simulink model "BG"  (R2014a)
settings: Solver=ode3  StartTime=0.0  StopTime=1  FixedStep=dt  MaxStep=dt  RelTol=1e-3
values from neighbouring files (symbols this model uses):
  a1 = .4    (= 0.4)    [parameters.m]
  a2 = .35    (= 0.35)    [parameters.m]
  a3 = .25    (= 0.25)    [parameters.m]
  aTc = 0.05    [parameters.m]
  dt = 1e-3    (= 0.001)    [parameters.m]
  g = 1    [parameters.m]
  K = 1    [parameters.m]
  mTc = 0.01    [parameters.m]
  OP1_0 = [ax1_0 ay1_0 0]    [parameters.m]
  OP2_0 = OP1_0 + P1P2_0    [parameters.m]
  OP3_0 = OP2_0 + P2P3_0    [parameters.m]
  OT = [xf yf 0]    [animation.m]    (also in parameters.m = [0.5 0.5 0])
  OT_cercle = [0.6 0.55 0]    [parameters.m]
  p1 = w2 + w3    (= 3)    [parameters.m]
  P1P2_0 = [ax2_0 ay2_0 0]    [parameters.m]
  p2 = w1 + w3    (= 4)    [parameters.m]
  P2P3_0 = [ax3_0 ay3_0 0]    [parameters.m]
  p3 = w2 + w1    (= 5)    [parameters.m]
  tau = 0.001    [parameters.m]
  theta1_0 = zero_vector    [parameters.m]
  theta2_0 = zero_vector    [parameters.m]
  theta3_0 = zero_vector    [parameters.m]
  Vmax = 30    [parameters.m]
  w1 = 3    [parameters.m]
  w2 = 2    [parameters.m]
  w3 = 1    [parameters.m]
  zero_vector = [0 0 0]    [parameters.m]
libraries: vrlib x9, simulink x1
(part 2 of 4)

== system BG/CNS/ Striosom//SNc2/Optimiseur1 ==
  v : Inport
  a1 : Inport  Port=2
  a2 : Inport  Port=3
  a3 : Inport  Port=4
  "                                                                                                    " : Sum  Inputs=+--
  B1 : Subsystem
  B2 : Subsystem
  Gain : Gain  Gain=w1
  Gain1 : Gain  Gain=w2
  Gamma1 : Subsystem
  Gamma2 : Subsystem
  lambda : Subsystem
  matrix_vector_multiplication : Subsystem
  matrix_vector_multiplication1 : Subsystem
  x : Scope
  v1 : Outport
  v2 : Outport  Port=2
  v3 : Outport  Port=3
  wires:
  v/1 -> "                                                                                                    "/1, matrix_vector_multiplication1/1(v1), matrix_vector_multiplication/1(v1), B2/1(v), B1/1(v), lambda/1(v)
  a1/1 -> B1/4(a1), lambda/2(a1)
  a2/1 -> B2/4(a2), lambda/3(a2)
  a3/1 -> B2/5(a3), B1/5(a3), lambda/4(a3)
  lambda/1(lambda1) -> B1/2(lambda1)
  lambda/3(lambda3) -> B1/3(lambda3), B2/3(lambda3)
  lambda/2(lamda2) -> B2/2(lambda2)
  B1/1(b11) -> Gamma2/5(b11_2), Gamma1/1(b11_1)
  B1/2(b12) -> Gamma2/6(b12_2), Gamma1/2(b12_1)
  B1/3(b21) -> Gamma2/7(b21_2), Gamma1/3(b21_1)
  B1/4(b22) -> Gamma2/8(b22_2), Gamma1/4(b22_1)
  B2/1(b11) -> Gamma1/5(b11_2), Gamma2/1(b11_1)
  B2/2(b12) -> Gamma1/6(b12_2), Gamma2/2(b12_1)
  B2/3(b21) -> Gamma1/7(b21_2), Gamma2/3(b21_1)
  B2/4(b22) -> Gamma2/4(b22_1), Gamma1/8(b22_2)
  Gamma1/1(gamma11) -> matrix_vector_multiplication/2(a11)
  Gamma1/2(gamma12) -> matrix_vector_multiplication/3(a12)
  Gamma1/3(gamma21) -> matrix_vector_multiplication/4(a21)
  Gamma1/4(gamma22) -> matrix_vector_multiplication/5(a22)
  Gamma2/1(gamma11) -> matrix_vector_multiplication1/2(a11)
  Gamma2/2(gamma12) -> matrix_vector_multiplication1/3(a12)
  Gamma2/3(gamma21) -> matrix_vector_multiplication1/4(a21)
  Gamma2/4(gamma22) -> matrix_vector_multiplication1/5(a22)
  matrix_vector_multiplication/1(vec_out) -> Gain/1
  matrix_vector_multiplication1/1(vec_out) -> Gain1/1
  "                                                                                                    "/1 -> v3/1
  Gain/1 -> x/1, "                                                                                                    "/2, v1/1
  Gain1/1 -> "                                                                                                    "/3, v2/1

== system BG/CNS/ Striosom//SNc2/derivative ==
  x : Inport
  Add : Sum  Inputs=+-
  Delay : Delay  DelayLength=1  InitialCondition=zero_vector
  Gain : Gain  Gain=1/dt
  z : Outport
  wires:
  Add/1 -> Gain/1
  x/1 -> Delay/1, Add/1
  Delay/1 -> Add/2
  Gain/1 -> z/1

== system BG/CNS/ Striosom//SNc2/derivative1 ==
  x : Inport
  Add : Sum  Inputs=+-
  Delay : Delay  DelayLength=1  InitialCondition=zero_vector
  Gain : Gain  Gain=1/dt
  z : Outport
  wires:
  Add/1 -> Gain/1
  x/1 -> Delay/1, Add/1
  Delay/1 -> Add/2
  Gain/1 -> z/1

== system BG/CNS/ Striosom//SNc2/derivative2 ==
  x : Inport
  Add : Sum  Inputs=+-
  Delay : Delay  DelayLength=1  InitialCondition=zero_vector
  Gain : Gain  Gain=1/dt
  z : Outport
  wires:
  Add/1 -> Gain/1
  x/1 -> Delay/1, Add/1
  Delay/1 -> Add/2
  Gain/1 -> z/1

== system BG/CNS/ Striosom//SNc2/vector_scope1 ==
  In_vec : Inport
  Demux : Demux  Outputs=3
  x : Scope
  y : Scope
      settings: SaveName=ScopeData2
  z : Scope
      settings: SaveName=ScopeData3
  wires:
  In_vec/1 -> Demux/1
  Demux/1 -> x/1
  Demux/2 -> y/1
  Demux/3 -> z/1

== system BG/CNS/ Striosom//SNc2/vector_scope2 ==
  In_vec : Inport
  Demux : Demux  Outputs=3
  x : Scope
  y : Scope
      settings: SaveName=ScopeData2
  z : Scope
      settings: SaveName=ScopeData3
  wires:
  In_vec/1 -> Demux/1
  Demux/1 -> x/1
  Demux/2 -> y/1
  Demux/3 -> z/1

== system BG/CNS/ Striosom//SNc2/vector_scope3 ==
  In_vec : Inport
  Demux : Demux  Outputs=3
  x : Scope
  y : Scope
      settings: SaveName=ScopeData2
  z : Scope
      settings: SaveName=ScopeData3
  wires:
  In_vec/1 -> Demux/1
  Demux/1 -> x/1
  Demux/2 -> y/1
  Demux/3 -> z/1

== system BG/CNS/Circular movement/1//(T*s+1) ==
  x : Inport
  Add : Sum  Inputs=+-
  Add1 : Sum
  Delay : Delay  DelayLength=1  InitialCondition=OP3_0
  Gain : Gain  Gain=dt
  Gain2 : Gain  Gain=1/0.01
  z : Outport
  wires:
  Add/1 -> Gain/1
  Delay/1 -> Add1/2, Add/2
  Gain/1 -> Gain2/1
  x/1 -> Add/1
  Add1/1 -> z/1, Delay/1
  Gain2/1 -> Add1/1

== system BG/CNS/Circular movement/1//(T*s+1)1 ==
  x : Inport
  Add : Sum  Inputs=+-
  Add1 : Sum
  Delay : Delay  DelayLength=1  InitialCondition=OP3_0
  Gain : Gain  Gain=dt
  Gain2 : Gain  Gain=1/0.001
  z : Outport
  wires:
  Add/1 -> Gain/1
  Delay/1 -> Add1/2, Add/2
  Gain/1 -> Gain2/1
  x/1 -> Add/1
  Add1/1 -> z/1, Delay/1
  Gain2/1 -> Add1/1

== system BG/CNS/Circular movement/1//(T*s+1)2 ==
  x : Inport
  Add : Sum  Inputs=+-
  Add1 : Sum
  Delay : Delay  DelayLength=1  InitialCondition=OP3_0
  Gain : Gain  Gain=dt
  Gain2 : Gain  Gain=1/0.002
  z : Outport
  wires:
  Add/1 -> Gain/1
  Delay/1 -> Add1/2, Add/2
  Gain/1 -> Gain2/1
  x/1 -> Add/1
  Add1/1 -> z/1, Delay/1
  Gain2/1 -> Add1/1

== system BG/CNS/Circular movement/Theta_point1 ==
  In_vec : Inport
  Demux : Demux  Outputs=3
  x : Scope
      settings: YMin=0.74125  YMax=0.745
  y : Scope
      settings: YMin=0.59325  YMax=0.5965  SaveName=ScopeData2
  z : Scope
      settings: SaveName=ScopeData3
  wires:
  In_vec/1 -> Demux/1
  Demux/2 -> y/1
  Demux/3 -> z/1
  Demux/1 -> x/1

== system BG/CNS/Circular movement/Theta_point2 ==
  In_vec : Inport
  Demux : Demux  Outputs=3
  x : Scope
      settings: YMin=0.74125  YMax=0.745
  y : Scope
      settings: YMin=0.45  YMax=0.75  SaveName=ScopeData2
  z : Scope
      settings: SaveName=ScopeData3
  wires:
  In_vec/1 -> Demux/1
  Demux/2 -> y/1
  Demux/3 -> z/1
  Demux/1 -> x/1

== system BG/CNS/Circular movement/Theta_point3 ==
  In_vec : Inport
  Demux : Demux  Outputs=3
  x : Scope
      settings: YMin=0.74125  YMax=0.745
  y : Scope
      settings: YMin=0.59325  YMax=0.5965  SaveName=ScopeData2
  z : Scope
      settings: SaveName=ScopeData3
  wires:
  In_vec/1 -> Demux/1
  Demux/2 -> y/1
  Demux/3 -> z/1
  Demux/1 -> x/1

== system BG/CNS/Cortex M1/derivative ==
  x : Inport
  Add : Sum  Inputs=+-
  Delay : Delay  DelayLength=1  InitialCondition=zero_vector
  Gain : Gain  Gain=1/dt
  z : Outport
  wires:
  Add/1 -> Gain/1
  x/1 -> Delay/1, Add/1
  Delay/1 -> Add/2
  Gain/1 -> z/1

== system BG/CNS/Cortex M1/derivative1 ==
  x : Inport
  Add : Sum  Inputs=+-
  Delay : Delay  DelayLength=1  InitialCondition=zero_vector
  Gain : Gain  Gain=1/dt
  z : Outport
  wires:
  Add/1 -> Gain/1
  x/1 -> Delay/1, Add/1
  Delay/1 -> Add/2
  Gain/1 -> z/1

== system BG/CNS/Cortex M1/derivative2 ==
  x : Inport
  Add : Sum  Inputs=+-
  Delay : Delay  DelayLength=1  InitialCondition=zero_vector
  Gain : Gain  Gain=1/dt
  z : Outport
  wires:
  Add/1 -> Gain/1
  x/1 -> Delay/1, Add/1
  Delay/1 -> Add/2
  Gain/1 -> z/1

== system BG/CNS/GPe/1//(sigma*s+1) ==
  x : Inport
  Add : Sum  Inputs=+-
  Add1 : Sum
  Delay : Delay  DelayLength=1  InitialCondition=zero_vector
  Gain : Gain  Gain=dt
  Gain1 : Gain  Gain=0.9999999
  Gain2 : Gain  Gain=1/tau
  z : Outport
  wires:
  Add/1 -> Gain/1
  Gain1/1 -> Add1/2, Add/2
  Delay/1 -> Gain1/1
  Gain/1 -> Gain2/1
  x/1 -> Add/1
  Add1/1 -> z/1, Delay/1
  Gain2/1 -> Add1/1

== system BG/CNS/GPe/1//(sigma*s+1)1 ==
  x : Inport
  Add : Sum  Inputs=+-
  Add1 : Sum
  Delay : Delay  DelayLength=1  InitialCondition=zero_vector
  Gain : Gain  Gain=dt
  Gain1 : Gain  Gain=0.9999999
  Gain2 : Gain  Gain=1/tau
  z : Outport
  wires:
  Add/1 -> Gain/1
  Gain1/1 -> Add1/2, Add/2
  Delay/1 -> Gain1/1
  Gain/1 -> Gain2/1
  x/1 -> Add/1
  Add1/1 -> z/1, Delay/1
  Gain2/1 -> Add1/1

== system BG/CNS/GPe/1//(sigma*s+1)2 ==
  x : Inport
  Add : Sum  Inputs=+-
  Add1 : Sum
  Delay : Delay  DelayLength=1  InitialCondition=zero_vector
  Gain : Gain  Gain=dt
  Gain1 : Gain  Gain=0.9999999
  Gain2 : Gain  Gain=1/tau
  z : Outport
  wires:
  Add/1 -> Gain/1
  Gain1/1 -> Add1/2, Add/2
  Delay/1 -> Gain1/1
  Gain/1 -> Gain2/1
  x/1 -> Add/1
  Add1/1 -> z/1, Delay/1
  Gain2/1 -> Add1/1

== system BG/CNS/GPe/Theta_point4 ==
  In_vec : Inport
  Demux : Demux  Outputs=3
  x : Scope
  y : Scope
      settings: SaveName=ScopeData2
  z : Scope
      settings: TimeRange=2  SaveName=ScopeData3
  wires:
  In_vec/1 -> Demux/1
  Demux/1 -> x/1
  Demux/2 -> y/1
  Demux/3 -> z/1

== system BG/CNS/Gains  (STR1)/Normaliser ==
  PS1 : Inport
  PS2 : Inport  Port=2
  PS3 : Inport  Port=3
  PV1 : Inport  Port=4
  PV2 : Inport  Port=5
  PV 3 : Inport  Port=6
  "                  " : Sum
  "                                  " : Gain  Gain=1/(a1^2)
  "                                       " : Sum
  "                                                                    " : Gain  Gain=1/(a2^2)
  "                                                                                     " : Sum
  "                                                                                                               " : Gain  Gain=1/(a3^2)
  PS1+PV1 : Outport
  PS2+PV2 : Outport  Port=2
  PS3+PV3 : Outport  Port=3
  wires:
  "                  "/1 -> "                                                                    "/1
  PV2/1 -> "                  "/2
  PS2/1 -> "                  "/1
  "                                                                    "/1 -> PS2+PV2/1
  "                                  "/1 -> PS1+PV1/1
  "                                                                                     "/1 -> "                                  "/1
  PV1/1 -> "                                                                                     "/2
  PS1/1 -> "                                                                                     "/1
  "                                       "/1 -> "                                                                                                               "/1
  "                                                                                                               "/1 -> PS3+PV3/1
  PV 3/1 -> "                                       "/2
  PS3/1 -> "                                       "/1

== system BG/CNS/Positionof segments Forward Kinematics/unit_vec ==
  vec1 : Inport
  Divide : Product  Inputs=*/
  Dot Product3 : DotProduct  InputSameDT=on  OutDataTypeStr=Inherit: Inherit via internal rule
  Sqrt : Sqrt  SaturateOnIntegerOverflow=on
  vec2 : Outport
  wires:
  vec1/1 -> Divide/1, Dot Product3/2, Dot Product3/1
  Dot Product3/1 -> Sqrt/1
  Sqrt/1 -> Divide/2
  Divide/1 -> vec2/1

== system BG/CNS/Positionof segments Forward Kinematics/unit_vec1 ==
  vec1 : Inport
  Divide : Product  Inputs=*/
  Dot Product3 : DotProduct  InputSameDT=on  OutDataTypeStr=Inherit: Inherit via internal rule
  Sqrt : Sqrt  SaturateOnIntegerOverflow=on
  vec2 : Outport
  wires:
  vec1/1 -> Divide/1, Dot Product3/2, Dot Product3/1
  Dot Product3/1 -> Sqrt/1
  Sqrt/1 -> Divide/2
  Divide/1 -> vec2/1

== system BG/CNS/Positionof segments Forward Kinematics/unit_vec2 ==
  vec1 : Inport
  Divide : Product  Inputs=*/
  Dot Product3 : DotProduct  InputSameDT=on  OutDataTypeStr=Inherit: Inherit via internal rule
  Sqrt : Sqrt  SaturateOnIntegerOverflow=on
  vec2 : Outport
  wires:
  vec1/1 -> Divide/1, Dot Product3/2, Dot Product3/1
  Dot Product3/1 -> Sqrt/1
  Sqrt/1 -> Divide/2
  Divide/1 -> vec2/1

== system BG/CNS/Reaching/1//(T*s+1) ==
  x : Inport
  Add : Sum  Inputs=+-
  Add1 : Sum
  Delay : Delay  DelayLength=1  InitialCondition=OP3_0
  Gain : Gain  Gain=dt
  Gain2 : Gain  Gain=1/0.01
  z : Outport
  wires:
  Add/1 -> Gain/1
  Delay/1 -> Add1/2, Add/2
  Gain/1 -> Gain2/1
  x/1 -> Add/1
  Add1/1 -> z/1, Delay/1
  Gain2/1 -> Add1/1

== system BG/CNS/Reaching/Theta_point1 ==
  In_vec : Inport
  Demux : Demux  Outputs=3
  x : Scope
  y : Scope
      settings: SaveName=ScopeData2
  z : Scope
      settings: SaveName=ScopeData3
  wires:
  In_vec/1 -> Demux/1
  Demux/1 -> x/1
  Demux/2 -> y/1
  Demux/3 -> z/1

== system BG/CNS/Reaching/derivative ==
  x : Inport
  Add : Sum  Inputs=+-
  Delay : Delay  DelayLength=1  InitialCondition=OP3_0
  Gain : Gain  Gain=1/dt
  z : Outport
  wires:
  Add/1 -> Gain/1
  x/1 -> Delay/1, Add/1
  Delay/1 -> Add/2
  Gain/1 -> z/1

== system BG/CNS/Reaching/vitesse ==
  In_vec : Inport
  Demux : Demux  Outputs=3
  x : Scope
      settings: TimeRange=1.4  YMin=-90  YMax=0
  y : Scope
      settings: SaveName=ScopeData2
  z : Scope
      settings: SaveName=ScopeData3
  wires:
  In_vec/1 -> Demux/1
  Demux/1 -> x/1
  Demux/2 -> y/1
  Demux/3 -> z/1

== system BG/CNS/STN/1//(sigma*s+1) ==
  x : Inport
  Add : Sum  Inputs=+-
  Add1 : Sum
  Delay : Delay  DelayLength=1  InitialCondition=0
  Gain : Gain  Gain=dt
  Gain1 : Gain  Gain=0.9999999
  Gain2 : Gain  Gain=1/mTc
  z : Outport
  wires:
  Add/1 -> Gain/1
  Gain1/1 -> Add1/2, Add/2
  Delay/1 -> Gain1/1
  Gain/1 -> Gain2/1
  x/1 -> Add/1
  Gain2/1 -> Add1/1
  Add1/1 -> z/1, Delay/1

== system BG/CNS/STN/1//(sigma*s+1)1 ==
  x : Inport
  Add : Sum  Inputs=+-
  Add1 : Sum
  Delay : Delay  DelayLength=1  InitialCondition=0
  Gain : Gain  Gain=dt
  Gain1 : Gain  Gain=0.9999999
  Gain2 : Gain  Gain=1/mTc
  z : Outport
  wires:
  Add/1 -> Gain/1
  Gain1/1 -> Add1/2, Add/2
  Delay/1 -> Gain1/1
  Gain/1 -> Gain2/1
  x/1 -> Add/1
  Gain2/1 -> Add1/1
  Add1/1 -> z/1, Delay/1

== system BG/CNS/STN/1//(sigma*s+1)2 ==
  x : Inport
  Add : Sum  Inputs=+-
  Add1 : Sum
  Delay : Delay  DelayLength=1  InitialCondition=0
  Gain : Gain  Gain=dt
  Gain1 : Gain  Gain=0.9999999
  Gain2 : Gain  Gain=1/mTc
  z : Outport
  wires:
  Add/1 -> Gain/1
  Gain1/1 -> Add1/2, Add/2
  Delay/1 -> Gain1/1
  Gain/1 -> Gain2/1
  x/1 -> Add/1
  Gain2/1 -> Add1/1
  Add1/1 -> z/1, Delay/1

== system BG/CNS/STN/s//(Ts+1) ==
  In1 : Inport
  1/(sigma*s+1) : Subsystem  TreatAsAtomicUnit=on
  derivative : Subsystem  TreatAsAtomicUnit=on
  Out1 : Outport
  wires:
  In1/1 -> 1/(sigma*s+1)/1(x)
  1/(sigma*s+1)/1(z) -> derivative/1(x)
  derivative/1(z) -> Out1/1

== system BG/CNS/STN/s//(Ts+1)2 ==
  In1 : Inport
  1/(sigma*s+1) : Subsystem  TreatAsAtomicUnit=on
  derivative : Subsystem  TreatAsAtomicUnit=on
  Out1 : Outport
  wires:
  In1/1 -> 1/(sigma*s+1)/1(x)
  1/(sigma*s+1)/1(z) -> derivative/1(x)
  derivative/1(z) -> Out1/1

== system BG/CNS/STN/s//(Ts+1)3 ==
  In1 : Inport
  1/(sigma*s+1) : Subsystem  TreatAsAtomicUnit=on
  derivative : Subsystem  TreatAsAtomicUnit=on
  Out1 : Outport
  wires:
  In1/1 -> 1/(sigma*s+1)/1(x)
  1/(sigma*s+1)/1(z) -> derivative/1(x)
  derivative/1(z) -> Out1/1

== system BG/CNS/Thalamus/Theta_point1 ==
  In_vec : Inport
  Demux : Demux  Outputs=3
  x : Scope
  y : Scope
      settings: SaveName=ScopeData2
  z : Scope
      settings: SaveName=ScopeData3
  wires:
  In_vec/1 -> Demux/1
  Demux/1 -> x/1
  Demux/2 -> y/1
  Demux/3 -> z/1

== system BG/CNS/Vector Product  (STR1)/Integrateur ==
  In1 : Inport
  " " : Delay  DelayLength=1  InitialCondition=zero_vector
  "  " : Sum
  "        " : Gain  Gain=dt
  Out1 : Outport
  wires:
  "        "/1 -> "  "/1
  " "/1 -> "  "/2
  In1/1 -> "        "/1
  "  "/1 -> " "/1, Out1/1

== system BG/CNS/Vector Product  (STR1)/Integrateur1 ==
  In1 : Inport
  " " : Delay  DelayLength=1  InitialCondition=zero_vector
  "  " : Sum
  "        " : Gain  Gain=dt
  Out1 : Outport
  wires:
  "        "/1 -> "  "/1
  " "/1 -> "  "/2
  In1/1 -> "        "/1
  "  "/1 -> " "/1, Out1/1

== system BG/CNS/Vector Product  (STR1)/Integrateur2 ==
  In1 : Inport
  " " : Delay  DelayLength=1  InitialCondition=zero_vector
  "  " : Sum
  "        " : Gain  Gain=dt
  Out1 : Outport
  wires:
  "        "/1 -> "  "/1
  " "/1 -> "  "/2
  In1/1 -> "        "/1
  "  "/1 -> " "/1, Out1/1

== system BG/CNS/ Striosom//SNc2/Optimiseur/B1 ==
  v : Inport
  lambda1 : Inport  Port=2
  lambda3 : Inport  Port=3
  a1 : Inport  Port=4
  a3 : Inport  Port=5
  Subsystem : Subsystem
  inverse_matrix : Subsystem
  vector_in_matrix_out : Subsystem
  b11 : Outport
  b12 : Outport  Port=2
  b21 : Outport  Port=3
  b22 : Outport  Port=4
  wires:
  vector_in_matrix_out/3(a21_out) -> inverse_matrix/3(a21)
  vector_in_matrix_out/1(a11_out) -> inverse_matrix/1(a11)
  vector_in_matrix_out/4(a22_out) -> inverse_matrix/4(a22)
  vector_in_matrix_out/2(a12_out) -> inverse_matrix/2(a12)
  lambda3/1 -> Subsystem/3(lambda3)
  inverse_matrix/3(a21_out) -> Subsystem/7(In7)
  a1/1 -> Subsystem/2(a1)
  a3/1 -> Subsystem/4(a3)
  v/1 -> vector_in_matrix_out/1(v1), vector_in_matrix_out/2(v2), Subsystem/8(In8)
  Subsystem/4(b22) -> b22/1
  Subsystem/3(b21) -> b21/1
  inverse_matrix/2(a12_out) -> Subsystem/6(In6)
  inverse_matrix/4(a22_out) -> Subsystem/9(In9)
  inverse_matrix/1(a11_out) -> Subsystem/5(In5)
  lambda1/1 -> Subsystem/1(lambda1)
  Subsystem/2(b12) -> b12/1
  Subsystem/1(b11) -> b11/1

== system BG/CNS/ Striosom//SNc2/Optimiseur/B2 ==
  v : Inport
  lambda2 : Inport  Port=2
  lambda3 : Inport  Port=3
  a2 : Inport  Port=4
  a3 : Inport  Port=5
  Subsystem : Subsystem
  inverse_matrix : Subsystem
  vector_in_matrix_out : Subsystem
  b11 : Outport
  b12 : Outport  Port=2
  b21 : Outport  Port=3
  b22 : Outport  Port=4
  wires:
  vector_in_matrix_out/3(a21_out) -> inverse_matrix/3(a21)
  vector_in_matrix_out/1(a11_out) -> inverse_matrix/1(a11)
  vector_in_matrix_out/4(a22_out) -> inverse_matrix/4(a22)
  vector_in_matrix_out/2(a12_out) -> inverse_matrix/2(a12)
  lambda3/1 -> Subsystem/3(lambda3)
  inverse_matrix/3(a21_out) -> Subsystem/7(In7)
  a2/1 -> Subsystem/2(a1)
  a3/1 -> Subsystem/4(a3)
  v/1 -> vector_in_matrix_out/1(v1), vector_in_matrix_out/2(v2), Subsystem/8(In8)
  Subsystem/4(b22) -> b22/1
  Subsystem/3(b21) -> b21/1
  inverse_matrix/2(a12_out) -> Subsystem/6(In6)
  inverse_matrix/4(a22_out) -> Subsystem/9(In9)
  inverse_matrix/1(a11_out) -> Subsystem/5(In5)
  lambda2/1 -> Subsystem/1(lambda1)
  Subsystem/2(b12) -> b12/1
  Subsystem/1(b11) -> b11/1

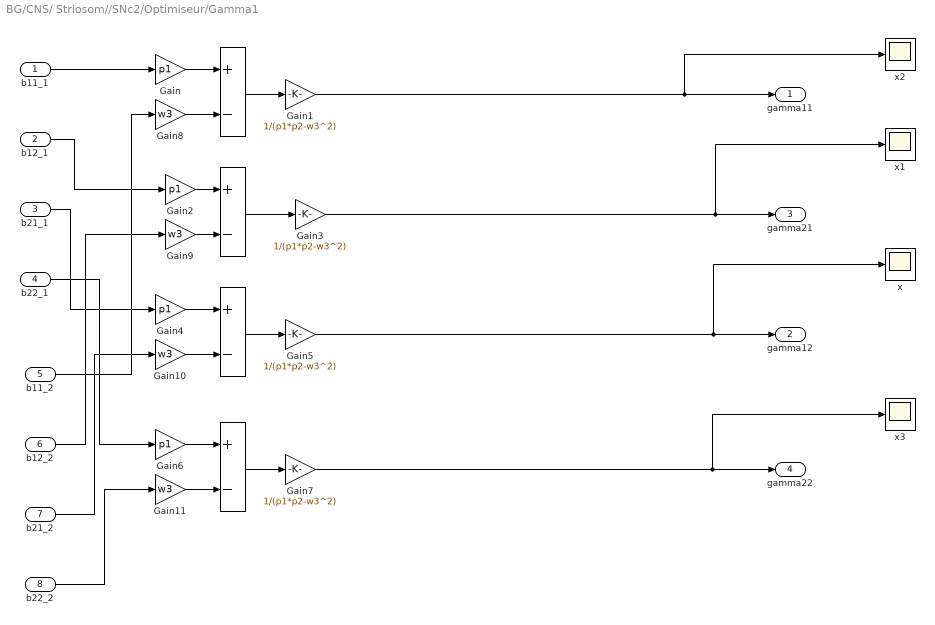
== system BG/CNS/ Striosom//SNc2/Optimiseur/Gamma1 ==
  b11_1 : Inport
  b12_1 : Inport  Port=2
  b21_1 : Inport  Port=3
  b22_1 : Inport  Port=4
  b11_2 : Inport  Port=5
  b12_2 : Inport  Port=6
  b21_2 : Inport  Port=7
  b22_2 : Inport  Port=8
  "                                                                                        " : Sum  Inputs=+-
  "                                                                                                " : Sum  Inputs=+-
  "                                                                                                  " : Sum  Inputs=+-
  "                                                                                                       " : Sum  Inputs=+-
  Gain{,2,4,6} (4 alike) : Gain  Gain=p1
  Gain{1,3,5,7} (4 alike) : Gain  Gain=1/(p1*p2-w3^2)
  Gain{8..11} (4 alike) : Gain  Gain=w3
  x{,1..3} (4 alike) : Scope
      x settings: YMin=-0.0001  YMax=0.0001  SaveName=ScopeData13
      x1 settings: YMin=-0.00045  YMax=0.0004  SaveName=ScopeData14
      x2 settings: YMin=-0.34905  YMax=-0.3486  SaveName=ScopeData15
      x3 settings: YMin=-0.348975  YMax=-0.348775  SaveName=ScopeData16
  gamma11 : Outport
  gamma12 : Outport  Port=2
  gamma21 : Outport  Port=3
  gamma22 : Outport  Port=4
  wires:
  b22_1/1 -> Gain6/1
  b21_1/1 -> Gain4/1
  b22_2/1 -> Gain11/1
  b11_1/1 -> Gain/1
  "                                                                                        "/1 -> Gain7/1
  "                                                                                                "/1 -> Gain5/1
  Gain6/1 -> "                                                                                        "/1
  Gain4/1 -> "                                                                                                "/1
  b21_2/1 -> Gain10/1
  b11_2/1 -> Gain8/1
  "                                                                                                       "/1 -> Gain1/1
  "                                                                                                  "/1 -> Gain3/1
  b12_2/1 -> Gain9/1
  Gain2/1 -> "                                                                                                  "/1
  b12_1/1 -> Gain2/1
  Gain/1 -> "                                                                                                       "/1
  Gain1/1 -> x2/1, gamma11/1
  Gain3/1 -> x1/1, gamma21/1
  Gain7/1 -> x3/1, gamma22/1
  Gain5/1 -> x/1, gamma12/1
  Gain8/1 -> "                                                                                                       "/2
  Gain9/1 -> "                                                                                                  "/2
  Gain10/1 -> "                                                                                                "/2
  Gain11/1 -> "                                                                                        "/2

== system BG/CNS/ Striosom//SNc2/Optimiseur/Gamma2 ==
  b11_1 : Inport
  b12_1 : Inport  Port=2
  b21_1 : Inport  Port=3
  b22_1 : Inport  Port=4
  b11_2 : Inport  Port=5
  b12_2 : Inport  Port=6
  b21_2 : Inport  Port=7
  b22_2 : Inport  Port=8
  "                                                                                        " : Sum
  "                                                                                                " : Sum
  "                                                                                                  " : Sum
  "                                                                                                       " : Sum
  Gain{1,3,5,8} (4 alike) : Gain  Gain=1/(w3*(p1*p2-w3^2))
  Gain{9..12} (4 alike) : Gain  Gain=w3*p2
  Gain{2,4,6..7} (4 alike) : Gain  Gain=(1-p1*p2)
  gamma11 : Outport
  gamma12 : Outport  Port=2
  gamma21 : Outport  Port=3
  gamma22 : Outport  Port=4
  wires:
  b22_1/1 -> Gain6/1
  b21_1/1 -> Gain4/1
  b22_2/1 -> Gain12/1
  b11_1/1 -> Gain7/1
  "                                                                                        "/1 -> Gain5/1
  "                                                                                                "/1 -> Gain8/1
  Gain6/1 -> "                                                                                        "/1
  Gain4/1 -> "                                                                                                "/1
  b21_2/1 -> Gain11/1
  b11_2/1 -> Gain9/1
  "                                                                                                       "/1 -> Gain1/1
  "                                                                                                  "/1 -> Gain3/1
  b12_2/1 -> Gain10/1
  Gain2/1 -> "                                                                                                  "/1
  b12_1/1 -> Gain2/1
  Gain7/1 -> "                                                                                                       "/1
  Gain1/1 -> gamma11/1
  Gain3/1 -> gamma21/1
  Gain5/1 -> gamma22/1
  Gain8/1 -> gamma12/1
  Gain9/1 -> "                                                                                                       "/2
  Gain10/1 -> "                                                                                                  "/2
  Gain11/1 -> "                                                                                                "/2
  Gain12/1 -> "                                                                                        "/2

== system BG/CNS/ Striosom//SNc2/Optimiseur/lambda ==
  v : Inport
  a1 : Inport  Port=2
  a2 : Inport  Port=3
  a3 : Inport  Port=4
  alpha : Subsystem
  d=V^T(VV^T)^-1V : Subsystem
  lambda : Subsystem
  other_aux_variables : Subsystem
  producing_dot_productions : Subsystem
  x : Scope
      settings: YMin=-0.7  YMax=1  SaveName=ScopeData12
  lambda1 : Outport
  lamda2 : Outport  Port=2
  lambda3 : Outport  Port=3
  wires:
  other_aux_variables/1(beta) -> lambda/1(beta)
  other_aux_variables/2(delta1) -> lambda/2(delta1)
  other_aux_variables/3(delta2) -> lambda/3(delta2)
  a2/1 -> producing_dot_productions/3(a2)
  producing_dot_productions/8(b23) -> lambda/8(b23), other_aux_variables/5(b23)
  a3/1 -> producing_dot_productions/4(a3)
  producing_dot_productions/9(b33) -> lambda/9(b33), other_aux_variables/6(b33)
  producing_dot_productions/6(b13) -> other_aux_variables/3(b13), lambda/7(b13)
  alpha/3(alpha3) -> lambda/6(alpha3), other_aux_variables/9(alpha3)
  producing_dot_productions/1(c1) -> alpha/2(c1)
  producing_dot_productions/5(b12) -> other_aux_variables/2(b12)
  v/1 -> producing_dot_productions/1(v), d=V^T(VV^T)^-1V/1(In1)
  other_aux_variables/5(gessi2) -> lambda/5(gessi2)
  producing_dot_productions/7(b22) -> other_aux_variables/4(b22)
  producing_dot_productions/4(b11) -> other_aux_variables/1(b11)
  alpha/2(alpha2) -> other_aux_variables/8(alpha2)
  alpha/1(alpha1) -> other_aux_variables/7(alpha1)
  other_aux_variables/4(gessi1) -> lambda/4(gessi1)
  producing_dot_productions/3(c3) -> alpha/4(c3)
  a1/1 -> producing_dot_productions/2(a1)
  d=V^T(VV^T)^-1V/1(d) -> alpha/1(d)
  producing_dot_productions/2(c2) -> alpha/3(c2)
  lambda/1(lambda1) -> lambda1/1
  lambda/3(lambda3) -> lambda3/1
  lambda/2(lambda2) -> lamda2/1

== system BG/CNS/ Striosom//SNc2/Optimiseur/matrix_vector_multiplication ==
  v1 : Inport
  a11 : Inport  Port=2
  a12 : Inport  Port=3
  a21 : Inport  Port=4
  a22 : Inport  Port=5
  "                                                                                                    " : Sum
  "                                                                                                           " : Sum
  Demux : Demux  Outputs=3
  Mux : Mux  Inputs=3
  a{1..4} (4 alike) : Product
  vec_out : Outport
  wires:
  v1/1 -> Demux/1
  a11/1 -> a1/2
  a12/1 -> a2/2
  a1/1 -> "                                                                                                    "/1
  a2/1 -> "                                                                                                    "/2
  "                                                                                                    "/1 -> Mux/1
  Demux/1 -> a3/1, a1/1
  a21/1 -> a3/2
  Demux/2 -> a4/1, a2/1
  a22/1 -> a4/2
  a3/1 -> "                                                                                                           "/1
  a4/1 -> "                                                                                                           "/2
  "                                                                                                           "/1 -> Mux/2
  Mux/1 -> vec_out/1

== system BG/CNS/ Striosom//SNc2/Optimiseur/matrix_vector_multiplication1 ==
  v1 : Inport
  a11 : Inport  Port=2
  a12 : Inport  Port=3
  a21 : Inport  Port=4
  a22 : Inport  Port=5
  "                                                                                                    " : Sum
  "                                                                                                           " : Sum
  Demux : Demux  Outputs=3
  Mux : Mux  Inputs=3
  a{1..4} (4 alike) : Product
  vec_out : Outport
  wires:
  v1/1 -> Demux/1
  a11/1 -> a1/2
  a12/1 -> a2/2
  a1/1 -> "                                                                                                    "/1
  a2/1 -> "                                                                                                    "/2
  "                                                                                                    "/1 -> Mux/1
  Demux/1 -> a3/1, a1/1
  a21/1 -> a3/2
  Demux/2 -> a4/1, a2/1
  a22/1 -> a4/2
  a3/1 -> "                                                                                                           "/1
  a4/1 -> "                                                                                                           "/2
  "                                                                                                           "/1 -> Mux/2
  Mux/1 -> vec_out/1

== system BG/CNS/ Striosom//SNc2/Optimiseur1/B1 ==
  v : Inport
  lambda1 : Inport  Port=2
  lambda3 : Inport  Port=3
  a1 : Inport  Port=4
  a3 : Inport  Port=5
  Subsystem : Subsystem
  inverse_matrix : Subsystem
  vector_in_matrix_out : Subsystem
  b11 : Outport
  b12 : Outport  Port=2
  b21 : Outport  Port=3
  b22 : Outport  Port=4
  wires:
  vector_in_matrix_out/3(a21_out) -> inverse_matrix/3(a21)
  vector_in_matrix_out/1(a11_out) -> inverse_matrix/1(a11)
  vector_in_matrix_out/4(a22_out) -> inverse_matrix/4(a22)
  vector_in_matrix_out/2(a12_out) -> inverse_matrix/2(a12)
  lambda3/1 -> Subsystem/3(lambda3)
  inverse_matrix/3(a21_out) -> Subsystem/7(In7)
  a1/1 -> Subsystem/2(a1)
  a3/1 -> Subsystem/4(a3)
  v/1 -> vector_in_matrix_out/1(v1), vector_in_matrix_out/2(v2), Subsystem/8(In8)
  Subsystem/4(b22) -> b22/1
  Subsystem/3(b21) -> b21/1
  inverse_matrix/2(a12_out) -> Subsystem/6(In6)
  inverse_matrix/4(a22_out) -> Subsystem/9(In9)
  inverse_matrix/1(a11_out) -> Subsystem/5(In5)
  lambda1/1 -> Subsystem/1(lambda1)
  Subsystem/2(b12) -> b12/1
  Subsystem/1(b11) -> b11/1

== system BG/CNS/ Striosom//SNc2/Optimiseur1/B2 ==
  v : Inport
  lambda2 : Inport  Port=2
  lambda3 : Inport  Port=3
  a2 : Inport  Port=4
  a3 : Inport  Port=5
  Subsystem : Subsystem
  inverse_matrix : Subsystem
  vector_in_matrix_out : Subsystem
  b11 : Outport
  b12 : Outport  Port=2
  b21 : Outport  Port=3
  b22 : Outport  Port=4
  wires:
  vector_in_matrix_out/3(a21_out) -> inverse_matrix/3(a21)
  vector_in_matrix_out/1(a11_out) -> inverse_matrix/1(a11)
  vector_in_matrix_out/4(a22_out) -> inverse_matrix/4(a22)
  vector_in_matrix_out/2(a12_out) -> inverse_matrix/2(a12)
  lambda3/1 -> Subsystem/3(lambda3)
  inverse_matrix/3(a21_out) -> Subsystem/7(In7)
  a2/1 -> Subsystem/2(a1)
  a3/1 -> Subsystem/4(a3)
  v/1 -> vector_in_matrix_out/1(v1), vector_in_matrix_out/2(v2), Subsystem/8(In8)
  Subsystem/4(b22) -> b22/1
  Subsystem/3(b21) -> b21/1
  inverse_matrix/2(a12_out) -> Subsystem/6(In6)
  inverse_matrix/4(a22_out) -> Subsystem/9(In9)
  inverse_matrix/1(a11_out) -> Subsystem/5(In5)
  lambda2/1 -> Subsystem/1(lambda1)
  Subsystem/2(b12) -> b12/1
  Subsystem/1(b11) -> b11/1

== system BG/CNS/ Striosom//SNc2/Optimiseur1/Gamma1 ==
  b11_1 : Inport
  b12_1 : Inport  Port=2
  b21_1 : Inport  Port=3
  b22_1 : Inport  Port=4
  b11_2 : Inport  Port=5
  b12_2 : Inport  Port=6
  b21_2 : Inport  Port=7
  b22_2 : Inport  Port=8
  "                                                                                        " : Sum  Inputs=+-
  "                                                                                                " : Sum  Inputs=+-
  "                                                                                                  " : Sum  Inputs=+-
  "                                                                                                       " : Sum  Inputs=+-
  Gain{,2,4,6} (4 alike) : Gain  Gain=2
  Gain{1,3,5,7} (4 alike) : Gain  Gain=1/3
  gamma11 : Outport
  gamma12 : Outport  Port=2
  gamma21 : Outport  Port=3
  gamma22 : Outport  Port=4
  wires:
  b22_1/1 -> Gain6/1
  b21_1/1 -> Gain4/1
  b22_2/1 -> "                                                                                        "/2
  b11_1/1 -> Gain/1
  "                                                                                        "/1 -> Gain7/1
  "                                                                                                "/1 -> Gain5/1
  Gain6/1 -> "                                                                                        "/1
  Gain4/1 -> "                                                                                                "/1
  b21_2/1 -> "                                                                                                "/2
  b11_2/1 -> "                                                                                                       "/2
  "                                                                                                       "/1 -> Gain1/1
  "                                                                                                  "/1 -> Gain3/1
  b12_2/1 -> "                                                                                                  "/2
  Gain2/1 -> "                                                                                                  "/1
  b12_1/1 -> Gain2/1
  Gain/1 -> "                                                                                                       "/1
  Gain1/1 -> gamma11/1
  Gain3/1 -> gamma21/1
  Gain7/1 -> gamma22/1
  Gain5/1 -> gamma12/1

== system BG/CNS/ Striosom//SNc2/Optimiseur1/Gamma2 ==
  b11_1 : Inport
  b12_1 : Inport  Port=2
  b21_1 : Inport  Port=3
  b22_1 : Inport  Port=4
  b11_2 : Inport  Port=5
  b12_2 : Inport  Port=6
  b21_2 : Inport  Port=7
  b22_2 : Inport  Port=8
  "                                                                                        " : Sum  Inputs=+-
  "                                                                                                " : Sum  Inputs=+-
  "                                                                                                  " : Sum  Inputs=+-
  "                                                                                                       " : Sum  Inputs=+-
  Gain{,2,4,6} (4 alike) : Gain  Gain=2
  Gain{1,3,5,7} (4 alike) : Gain  Gain=1/3
  gamma11 : Outport
  gamma12 : Outport  Port=2
  gamma21 : Outport  Port=3
  gamma22 : Outport  Port=4
  wires:
  b22_1/1 -> Gain6/1
  b21_1/1 -> Gain4/1
  b22_2/1 -> "                                                                                        "/2
  b11_1/1 -> Gain/1
  "                                                                                        "/1 -> Gain7/1
  "                                                                                                "/1 -> Gain5/1
  Gain6/1 -> "                                                                                        "/1
  Gain4/1 -> "                                                                                                "/1
  b21_2/1 -> "                                                                                                "/2
  b11_2/1 -> "                                                                                                       "/2
  "                                                                                                       "/1 -> Gain1/1
  "                                                                                                  "/1 -> Gain3/1
  b12_2/1 -> "                                                                                                  "/2
  Gain2/1 -> "                                                                                                  "/1
  b12_1/1 -> Gain2/1
  Gain/1 -> "                                                                                                       "/1
  Gain1/1 -> gamma11/1
  Gain3/1 -> gamma21/1
  Gain7/1 -> gamma22/1
  Gain5/1 -> gamma12/1

== system BG/CNS/ Striosom//SNc2/Optimiseur1/lambda ==
  v : Inport
  a1 : Inport  Port=2
  a2 : Inport  Port=3
  a3 : Inport  Port=4
  alpha : Subsystem
  d=V^T(VV^T)^-1V : Subsystem
  lambda : Subsystem
  other_aux_variables : Subsystem
  producing_dot_productions : Subsystem
  lambda1 : Outport
  lamda2 : Outport  Port=2
  lambda3 : Outport  Port=3
  wires:
  other_aux_variables/1(beta) -> lambda/1(beta)
  other_aux_variables/2(delta1) -> lambda/2(delta1)
  other_aux_variables/3(delta2) -> lambda/3(delta2)
  a2/1 -> producing_dot_productions/3(a2)
  producing_dot_productions/8(b23) -> lambda/8(b23), other_aux_variables/5(b23)
  a3/1 -> producing_dot_productions/4(a3)
  producing_dot_productions/9(b33) -> lambda/9(b33), other_aux_variables/6(b33)
  producing_dot_productions/6(b13) -> other_aux_variables/3(b13), lambda/7(b13)
  alpha/3(alpha3) -> lambda/6(alpha3), other_aux_variables/9(alpha3)
  producing_dot_productions/1(c1) -> alpha/2(c1)
  producing_dot_productions/5(b12) -> other_aux_variables/2(b12)
  v/1 -> producing_dot_productions/1(v), d=V^T(VV^T)^-1V/1(In1)
  other_aux_variables/5(gessi2) -> lambda/5(gessi2)
  producing_dot_productions/7(b22) -> other_aux_variables/4(b22)
  producing_dot_productions/4(b11) -> other_aux_variables/1(b11)
  alpha/2(alpha2) -> other_aux_variables/8(alpha2)
  alpha/1(alpha1) -> other_aux_variables/7(alpha1)
  other_aux_variables/4(gessi1) -> lambda/4(gessi1)
  producing_dot_productions/3(c3) -> alpha/4(c3)
  a1/1 -> producing_dot_productions/2(a1)
  d=V^T(VV^T)^-1V/1(d) -> alpha/1(d)
  producing_dot_productions/2(c2) -> alpha/3(c2)
  lambda/1(lambda1) -> lambda1/1
  lambda/3(lambda3) -> lambda3/1
  lambda/2(lambda2) -> lamda2/1

== system BG/CNS/ Striosom//SNc2/Optimiseur1/matrix_vector_multiplication ==
  v1 : Inport
  a11 : Inport  Port=2
  a12 : Inport  Port=3
  a21 : Inport  Port=4
  a22 : Inport  Port=5
  "                                                                                                    " : Sum
  "                                                                                                           " : Sum
  Demux : Demux  Outputs=3
  Mux : Mux  Inputs=3
  a{1..4} (4 alike) : Product
  vec_out : Outport
  wires:
  v1/1 -> Demux/1
  a11/1 -> a1/2
  a12/1 -> a2/2
  a1/1 -> "                                                                                                    "/1
  a2/1 -> "                                                                                                    "/2
  "                                                                                                    "/1 -> Mux/1
  Demux/1 -> a3/1, a1/1
  a21/1 -> a3/2
  Demux/2 -> a4/1, a2/1
  a22/1 -> a4/2
  a3/1 -> "                                                                                                           "/1
  a4/1 -> "                                                                                                           "/2
  "                                                                                                           "/1 -> Mux/2
  Mux/1 -> vec_out/1

== system BG/CNS/ Striosom//SNc2/Optimiseur1/matrix_vector_multiplication1 ==
  v1 : Inport
  a11 : Inport  Port=2
  a12 : Inport  Port=3
  a21 : Inport  Port=4
  a22 : Inport  Port=5
  "                                                                                                    " : Sum
  "                                                                                                           " : Sum
  Demux : Demux  Outputs=3
  Mux : Mux  Inputs=3
  a{1..4} (4 alike) : Product
  vec_out : Outport
  wires:
  v1/1 -> Demux/1
  a11/1 -> a1/2
  a12/1 -> a2/2
  a1/1 -> "                                                                                                    "/1
  a2/1 -> "                                                                                                    "/2
  "                                                                                                    "/1 -> Mux/1
  Demux/1 -> a3/1, a1/1
  a21/1 -> a3/2
  Demux/2 -> a4/1, a2/1
  a22/1 -> a4/2
  a3/1 -> "                                                                                                           "/1
  a4/1 -> "                                                                                                           "/2
  "                                                                                                           "/1 -> Mux/2
  Mux/1 -> vec_out/1

== system BG/CNS/STN/s//(Ts+1)/1//(sigma*s+1) ==
  x : Inport
  Add : Sum  Inputs=+-
  Add1 : Sum
  Delay : Delay  DelayLength=1  InitialCondition=zero_vector
  Gain : Gain  Gain=dt
  Gain1 : Gain  Gain=0.9999999
  Gain2 : Gain  Gain=1/(aTc)
  z : Outport
  wires:
  Add/1 -> Gain/1
  Gain1/1 -> Add1/2, Add/2
  Delay/1 -> Gain1/1
  Gain/1 -> Gain2/1
  x/1 -> Add/1
  Add1/1 -> z/1, Delay/1
  Gain2/1 -> Add1/1

== system BG/CNS/STN/s//(Ts+1)/derivative ==
  x : Inport
  Add : Sum  Inputs=+-
  Delay : Delay  DelayLength=1  InitialCondition=zero_vector
  Gain : Gain  Gain=1/dt
  z : Outport
  wires:
  Add/1 -> Gain/1
  x/1 -> Delay/1, Add/1
  Delay/1 -> Add/2
  Gain/1 -> z/1

== system BG/CNS/STN/s//(Ts+1)2/1//(sigma*s+1) ==
  x : Inport
  Add : Sum  Inputs=+-
  Add1 : Sum
  Delay : Delay  DelayLength=1  InitialCondition=zero_vector
  Gain : Gain  Gain=dt
  Gain1 : Gain  Gain=0.9999999
  Gain2 : Gain  Gain=1/(aTc)
  z : Outport
  wires:
  Add/1 -> Gain/1
  Gain1/1 -> Add1/2, Add/2
  Delay/1 -> Gain1/1
  Gain/1 -> Gain2/1
  x/1 -> Add/1
  Add1/1 -> z/1, Delay/1
  Gain2/1 -> Add1/1

== system BG/CNS/STN/s//(Ts+1)2/derivative ==
  x : Inport
  Add : Sum  Inputs=+-
  Delay : Delay  DelayLength=1  InitialCondition=zero_vector
  Gain : Gain  Gain=1/dt
  z : Outport
  wires:
  Add/1 -> Gain/1
  x/1 -> Delay/1, Add/1
  Delay/1 -> Add/2
  Gain/1 -> z/1

== system BG/CNS/STN/s//(Ts+1)3/1//(sigma*s+1) ==
  x : Inport
  Add : Sum  Inputs=+-
  Add1 : Sum
  Delay : Delay  DelayLength=1  InitialCondition=zero_vector
  Gain : Gain  Gain=dt
  Gain1 : Gain  Gain=0.9999999
  Gain2 : Gain  Gain=1/(aTc)
  z : Outport
  wires:
  Add/1 -> Gain/1
  Gain1/1 -> Add1/2, Add/2
  Delay/1 -> Gain1/1
  Gain/1 -> Gain2/1
  x/1 -> Add/1
  Add1/1 -> z/1, Delay/1
  Gain2/1 -> Add1/1

== system BG/CNS/STN/s//(Ts+1)3/derivative ==
  x : Inport
  Add : Sum  Inputs=+-
  Delay : Delay  DelayLength=1  InitialCondition=zero_vector
  Gain : Gain  Gain=1/dt
  z : Outport
  wires:
  Add/1 -> Gain/1
  x/1 -> Delay/1, Add/1
  Delay/1 -> Add/2
  Gain/1 -> z/1

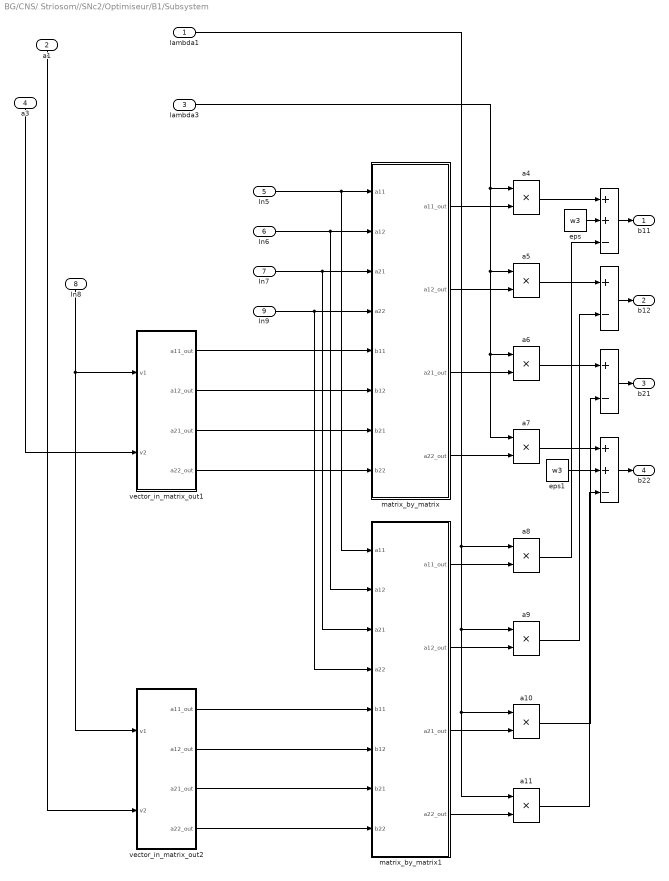
== system BG/CNS/ Striosom//SNc2/Optimiseur/B1/Subsystem ==
  lambda1 : Inport
  a1 : Inport  Port=2
  lambda3 : Inport  Port=3
  a3 : Inport  Port=4
  In5 : Inport  Port=5
  In6 : Inport  Port=6
  In7 : Inport  Port=7
  In8 : Inport  Port=8
  In9 : Inport  Port=9
  "                                                                                                    " : Sum  Inputs=++-
  "                                                                                                      " : Sum  Inputs=++-
  "                                                                                                       " : Sum  Inputs=+-
  "                                                                                                           " : Sum  Inputs=+-
  a{4..11} (8 alike) : Product
  eps : Constant  Value=w3
  eps1 : Constant  Value=w3
  matrix_by_matrix : Subsystem
  matrix_by_matrix1 : Subsystem
  vector_in_matrix_out1 : Subsystem
  vector_in_matrix_out2 : Subsystem
  b11 : Outport
  b12 : Outport  Port=2
  b21 : Outport  Port=3
  b22 : Outport  Port=4
  wires:
  In5/1 -> matrix_by_matrix1/1(a11), matrix_by_matrix/1(a11)
  In6/1 -> matrix_by_matrix1/2(a12), matrix_by_matrix/2(a12)
  In7/1 -> matrix_by_matrix1/3(a21), matrix_by_matrix/3(a21)
  In9/1 -> matrix_by_matrix1/4(a22), matrix_by_matrix/4(a22)
  vector_in_matrix_out1/4(a22_out) -> matrix_by_matrix/8(b22)
  vector_in_matrix_out1/3(a21_out) -> matrix_by_matrix/7(b21)
  vector_in_matrix_out1/1(a11_out) -> matrix_by_matrix/5(b11)
  vector_in_matrix_out1/2(a12_out) -> matrix_by_matrix/6(b12)
  matrix_by_matrix/1(a11_out) -> a4/2
  lambda3/1 -> a7/1, a6/1, a5/1, a4/1
  matrix_by_matrix/2(a12_out) -> a5/2
  matrix_by_matrix/3(a21_out) -> a6/2
  matrix_by_matrix/4(a22_out) -> a7/2
  vector_in_matrix_out2/2(a12_out) -> matrix_by_matrix1/6(b12)
  vector_in_matrix_out2/3(a21_out) -> matrix_by_matrix1/7(b21)
  vector_in_matrix_out2/1(a11_out) -> matrix_by_matrix1/5(b11)
  vector_in_matrix_out2/4(a22_out) -> matrix_by_matrix1/8(b22)
  matrix_by_matrix1/1(a11_out) -> a8/2
  matrix_by_matrix1/2(a12_out) -> a9/2
  matrix_by_matrix1/3(a21_out) -> a10/2
  matrix_by_matrix1/4(a22_out) -> a11/2
  lambda1/1 -> a11/1, a10/1, a9/1, a8/1
  a4/1 -> "                                                                                                    "/1
  a8/1 -> "                                                                                                    "/3
  eps/1 -> "                                                                                                    "/2
  a5/1 -> "                                                                                                       "/1
  a9/1 -> "                                                                                                       "/2
  a6/1 -> "                                                                                                           "/1
  a10/1 -> "                                                                                                           "/2
  a7/1 -> "                                                                                                      "/1
  eps1/1 -> "                                                                                                      "/2
  a11/1 -> "                                                                                                      "/3
  a1/1 -> vector_in_matrix_out2/2(v2)
  "                                                                                                       "/1 -> b12/1
  "                                                                                                           "/1 -> b21/1
  a3/1 -> vector_in_matrix_out1/2(v2)
  "                                                                                                      "/1 -> b22/1
  "                                                                                                    "/1 -> b11/1
  In8/1 -> vector_in_matrix_out2/1(v1), vector_in_matrix_out1/1(v1)

== system BG/CNS/ Striosom//SNc2/Optimiseur/B1/inverse_matrix ==
  a11 : Inport
  a12 : Inport  Port=2
  a21 : Inport  Port=3
  a22 : Inport  Port=4
  "                                                                                                    " : Sum  Inputs=+-+
  Divide{1..4} (4 alike) : Product  Inputs=*/
  Gain : Gain  Gain=-1
  Gain1 : Gain  Gain=-1
  a1 : Product
  a2 : Product
  eps : Constant  Value=1e-1
  a11_out : Outport
  a12_out : Outport  Port=2
  a21_out : Outport  Port=3
  a22_out : Outport  Port=4
  wires:
  a11/1 -> Divide2/1, a1/1
  a22/1 -> Divide1/1, a1/2
  a12/1 -> a2/1, Gain1/1
  a21/1 -> Gain/1, a2/2
  a1/1 -> "                                                                                                    "/1
  a2/1 -> "                                                                                                    "/2
  "                                                                                                    "/1 -> Divide1/2, Divide2/2, Divide3/2, Divide4/2
  Divide1/1 -> a11_out/1
  Divide2/1 -> a22_out/1
  Divide3/1 -> a12_out/1
  Divide4/1 -> a21_out/1
  Gain/1 -> Divide4/1
  Gain1/1 -> Divide3/1
  eps/1 -> "                                                                                                    "/3

== system BG/CNS/ Striosom//SNc2/Optimiseur/B1/vector_in_matrix_out ==
  v1 : Inport
  v2 : Inport  Port=2
  Demux : Demux  Outputs=3
  Demux1 : Demux  Outputs=3
  a{11..12,21..22} (4 alike) : Product
  a11_out : Outport
  a12_out : Outport  Port=2
  a21_out : Outport  Port=3
  a22_out : Outport  Port=4
  wires:
  v1/1 -> Demux/1
  v2/1 -> Demux1/1
  a11/1 -> a11_out/1
  Demux/1 -> a12/1, a11/1
  a12/1 -> a12_out/1
  a21/1 -> a21_out/1
  Demux/2 -> a22/1, a21/1
  a22/1 -> a22_out/1
  Demux1/1 -> a11/2, a21/2
  Demux1/2 -> a22/2, a12/2
